simulink model "PosControl_HIL_advanced"  (R2023b)
settings: Solver=FixedStepDiscrete  StartTime=0.0  StopTime=10.0  FixedStep=0.001  RelTol=1e-3
InitFcn:
  | Init_control
values from neighbouring files (symbols this model uses):
  DEG2RAD = 0.0174533    [Init_control.m]
  MAX_CONTROL_ANGLE_RATE_PITCH = 220    [Init_control.m]
  MAX_CONTROL_ANGLE_RATE_ROLL = 220    [Init_control.m]
  MAX_CONTROL_VELOCITY_XY = 5    [Init_control.m]
  MAX_CONTROL_VELOCITY_Z = 3    [Init_control.m]
  Saturation_I_az = 5    [Init_control.m]
undefined symbols (not defined in the file or in its folder): DiscIntNeverNeededParam
libraries: simulink x7, pixhawk_slib_uORB_RW x5, pixhawk_slib_sensors_actuators x4
(part 1 of 2)
settings Model: Creator=wsh  LastModifiedBy=02
settings SolverCC: AlgebraicLoopSolver=TrustRegion
settings DataIOCC: ReturnWorkspaceOutputs=off
settings OptimizationCC: DefaultParameterBehavior=Inlined  MaxStackSize=64  EfficientTunableParamExpr=on
settings DebuggingCC: ParameterTunabilityLossMsg=error  UnconnectedInputMsg=warning  UnconnectedOutputMsg=warning  UnconnectedLineMsg=warning  ArithmeticOperatorsInVariantConditions=warning
settings HardwareCC: ProdBitPerPointer=32  ProdBitPerSizeT=32  ProdBitPerPtrDiffT=32  ProdLargestAtomicInteger=Long  ProdLargestAtomicFloat=Double  ProdWordSize=32  ProdHWDeviceType=ARM Compatible->ARM Cortex
settings ModelReferenceCC: EnableRefExpFcnMdlSchedulingChecks=on
settings SFSimCC: SimUseLocalCustomCode=off  MATLABDynamicMemAlloc=off  CustomCodeUndefinedFunction=UseInterfaceOnly
settings RTWCC: Description=Embedded Coder  SystemTargetFile=ert.tlc  HardwareBoard=Pixhawk PX4  TLCOptions="-aInlineSetEventsForThisBaseRateFcn=TLC_FALSE -aSuppressMultiTaskScheduler=TLC_FALSE  -aRateBasedStepFcn=0"  TemplateMakefile=ert_default_tmf  GenerateReport=on  RTWUseLocalCustomCode=off  Toolchain=Pixhawk Toolchain  IncludeHyperlinkInReport=on  LaunchReport=on  GenerateTraceInfo=on  GenerateTraceReport=on  GenerateTraceReportSl=on  GenerateTraceReportSf=on  GenerateTraceReportEml=on
settings CodeAppCC: ForceParamTrailComments=on  IgnoreCustomStorageClasses=off  OperatorAnnotations=on  SimulinkDataObjDesc=on  SFDataObjDesc=on  MATLABFcnDesc=on  InsertBlockDesc=on  StateflowObjectComments=on  MATLABSourceComments=on
settings ERTTargetCC: MultiwordLength=2048  ERTCustomFileTemplate=PX4_codertarget_file_process.tlc

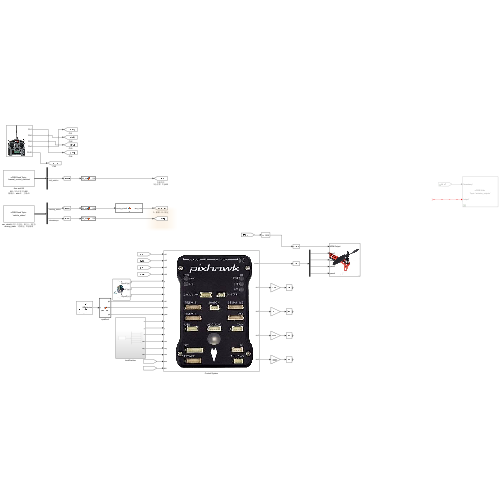
[thumbnail: Simulink's stored preview of the top-level diagram]
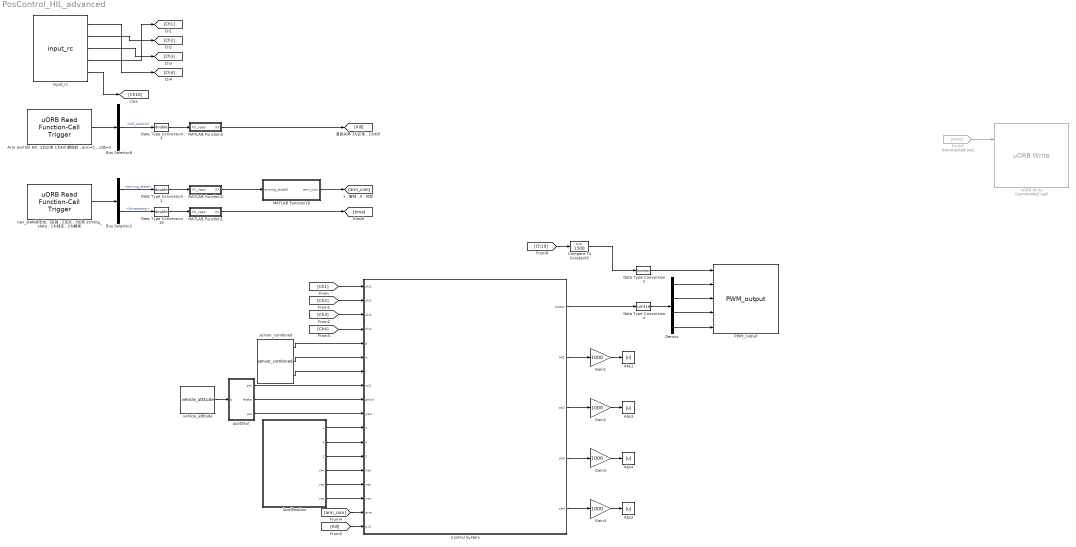
== system PosControl_HIL_advanced ==
  Abs{1..4} (4 alike) : Abs  SaturateOnIntegerOverflow=off
  Arm and Kill Kill：3为正常,1为Kill 解锁后，arm=1，上锁=3 : pixhawk_slib_uORB_RW/uORB Read Function-Call Trigger  uORB_Topic_str='manual_control_switches'  BusObjVar=Bus: manual_control_switches_SL  uORB_Interval=1  AsyncOutput=off  Fcn_call_select=Generate Function Call Signal  TaskName='Task1'  Poll_timeout=100  Ts=0.004
      settings: SourceProductName=Pixhawk Target Blocks
  Bus Selector2 : BusSelector  OutputSignals=arming_state,timestamp
  Bus Selector8 : BusSelector  OutputSignals=kill_switch
  Compare To Constant3 : simulink/Logic and Bit Operations/Compare To Constant  relop=>=  const=1500  OutDataTypeStr=boolean
  Control System : Subsystem
      mask Display: image('.\icon\pixhawk.png');
  Data Type Conversion1 : DataTypeConversion  OutDataTypeStr=double  SaturateOnIntegerOverflow=off  RndMeth=Floor
  Data Type Conversion19 : DataTypeConversion  OutDataTypeStr=double  SaturateOnIntegerOverflow=off  RndMeth=Floor
  Data Type Conversion2 : DataTypeConversion  OutDataTypeStr=boolean  SaturateOnIntegerOverflow=off  RndMeth=Floor
  Data Type Conversion3 : DataTypeConversion  OutDataTypeStr=double  SaturateOnIntegerOverflow=off  RndMeth=Floor
  Data Type Conversion4 : DataTypeConversion  OutDataTypeStr=uint16  SaturateOnIntegerOverflow=off  RndMeth=Floor
  Demux : Demux
  From6 : From  Commented=on  GotoTag=time
  Gain{1..4} (4 alike) : Gain  Gain=1000
  MATLAB Function1 : MATLAB Function  TreatAsAtomicUnit=on
  MATLAB Function18 : MATLAB Function  TreatAsAtomicUnit=on
  MATLAB Function2 : MATLAB Function  TreatAsAtomicUnit=on
  MATLAB Function3 : MATLAB Function  TreatAsAtomicUnit=on
  PWM_output : pixhawk_slib_sensors_actuators/PWM_output  Description=|  pub_outputs=on  pwm_rate=400Hz  show_pwm1=on  show_pwm5=off  show_pwm2=on  show_pwm6=off  show_pwm3=on  show_pwm7=off  show_pwm4=on  show_pwm8=off
      | This block allows the user to send the appropriate PWM signals out to the PX4 outputs.  
      | These are usually connected to the ESCs which control the motor speeds. 
      | In order for the flight control to arm (enable) the output from the software side, the ARM Output input must be held high (boolean TRUE).  
      | Only then will the PWM values be sent out the PX4 hardware ports.  
      | This is usually a function of the RC Tx in combination with other flight modes programmed in the Simulink model by the user.  
      | The block has 8 available ports (data type uint16) which can be selectively chosen.  
      | These correspond to the 8 PWM output ports on the px4fmu hardware.
      settings: SourceProductName=Pixhawk Target Blocks
  input_rc : pixhawk_slib_sensors_actuators/input_rc  Description=|  sampletime=0.004  channel1=on  channel2=on  channel3=on  channel4=on  channel5=off  channel6=off  channel7=off  channel8=off  channel9=off  channel10=on  channel11=off  channel12=off  channel13=off  channel14=off  channel15=off  channel16=off  channel17=off  channel18=off  ch_count=off  rssi=off  rc_failsafe=off  rc_lost=off  rc_inputsource=off
      | RC Input Block
      | 
      | This block provides user input control to the model.
      | It uses the input_rc uORB topic.
      | 
      | The user has the ability to choose which channels are available as outputs from this block and also some optional outputs. These include 
      | Channels 1 through 18
      | double data type indicating the PWM value from the controller 
      | measured pulse widths for each of the supported channels 
      | Channel Count 
      | uint32 data type of the number of channels which are detector by the PX4 
      | RC Failsafe 
      | boolean data types indicating that the RC Tx is sending the FailSafe signal (if equipped and properly setup) 
      | explicit failsafe flag: true on TX failure or TX out of range , false otherwise. 
      | Only the true state is reliable, as there are some (PPM) receivers on the market going into failsafe without telling us explicitly. 
      | RC Input Source 
      | Enumeration data type indicating which source the RC input is from. 
      | Valid values are found in the ENUM file: RC_INPUT_SOURCE_ENUM.m 
      |           Enumeration members for class 'RC_INPUT_SOURCE_ENUM':
      |           RCINPUT_SOURCE_UNKNOWN         (0)
      |           RCINPUT_SOURCE_PX4FMU_PPM      (1)
      |           RCINPUT_SOURCE_PX4IO_PPM       (2)
      |           RCINPUT_SOURCE_PX4IO_SPEKTRUM  (3)
      |           RCINPUT_SOURCE_PX4IO_SBUS      (4)
      |           RCINPUT_SOURCE_PX4IO_ST24      (5)
      |           RCINPUT_SOURCE_MAVLINK         (6)
      |           RCINPUT_SOURCE_QURT            (7)
      |           RCINPUT_SOURCE_PX4FMU_SPEKTRUM (8)
      |           RCINPUT_SOURCE_PX4FMU_SBUS     (9)
      |           RCINPUT_SOURCE_PX4FMU_ST24     (10)
      |           RCINPUT_SOURCE_PX4FMU_SUMD     (11)
      |           RCINPUT_SOURCE_PX4FMU_DSM      (12)
      |           RCINPUT_SOURCE_PX4IO_SUMD      (13)
      | 
      | RSSI - Receive signal strength index 
      | receive signal strength indicator (RSSI): < 0: Undefined, 0: no signal, 255: full reception 
      | RC Lost Connection 
      | boolean data type indicating RC receiver connection status 
      | True, if no frame has arrived in the expected time, false otherwise. 
      | True usally means that the receiver has been disconnected, but can also indicate a radio link loss on "stupid" systems. 
      | Will remain false, if a RX with failsafe option continues to transmit frames after a link loss. 
      |   
      | Sample Model: px4demo_input_rc.slx
      settings: SourceProductName=Pixhawk Target Blocks
  "localPosition " : Subsystem
  nav_state标志位: 1定高，2定点，3任务 arming_state：1为锁定，2为解锁 : pixhawk_slib_uORB_RW/uORB Read Function-Call Trigger  uORB_Topic_str='vehicle_status'  BusObjVar=Bus: vehicle_status_SL  uORB_Interval=1  AsyncOutput=off  Fcn_call_select=Generate Function Call Signal  TaskName='Task1'  Poll_timeout=100  Ts=0.004
      settings: SourceProductName=Pixhawk Target Blocks
  quat2eul : MATLAB Function  TreatAsAtomicUnit=on
  sensor_combined : pixhawk_slib_sensors_actuators/sensor_combined  Description=|  sampletime=0.001  show_mag=off  show_acc=off  show_gyro=on  show_baro=off  show_ts=off
      | Sensor Combined Block
      | 
      | This block enables access to the various sensors available on the px4fmu-v2 hardware.  
      | The user can use these signals in the Simulink control model.  
      | The sample time needs to be provided in the mask dialog.  
      | Optional output ports can also be selected.  
      | Refer to the sample model: px4demo_attitude_control.slx
      | 
      | Signal definitions: 
      | Magnetometer (x,y,z) - single values – Magnetic field in NED body frame, in Gauss 
      | Accelerometer (x,y,z) - single values – Acceleration in NED body frame, in m/s^2 
      | Gyroscope (p,q,r) - single values – Angular velocity in radians per second 
      | Barometer (Altitude) - single value – Barometric pressure, already temperature compensated (millibars) 
      | RunTime (timestamp) - double value – Timestamp in microseconds since boot, from gyro 
      |   
      | The sensor_combined block needs to have the px4io service running on the PX4 hardware in order to get valid signal values.
      settings: SourceProductName=Pixhawk Target Blocks
  uORB Write : pixhawk_slib_uORB_RW/uORB Write  Commented=on  uORB_Topic_str='actuator_outputs'  BlockOutputCount=2  OutputBoolean_1=on  uORB_Param_Name1='timestamp'  uORB_Param_Name_DT1=double  VectorScalar_1=1  OutputBoolean_2=on  uORB_Param_Name2='output'  uORB_Param_Name_DT2=double  VectorScalar_2=16  OutputBoolean_3=off  uORB_Param_Name3='timestamp_time'  uORB_Param_Name_DT3=double  VectorScalar_3=1  OutputBoolean_4=off  uORB_Param_Name4='gyro_temp'  uORB_Param_Name_DT4=single  VectorScalar_4=3  OutputBoolean_5=off  uORB_Param_Name5='vel_ned_valid'  uORB_Param_Name_DT5=boolean  VectorScalar_5=1  Ts=-1  MsgSizeOf=0
      settings: SourceProductName=Pixhawk Target Blocks
  vehicle_attitude : pixhawk_slib_sensors_actuators/vehicle_attitude  Description=|  sampletime=0.001  show_r=off  show_p=off  show_y=off  show_q=on  show_ts=off
      | This block gives access to the running service that calculates the vehicle’s attitude.  A uORB topic (vehicle_attitude (attitude measurements)) publisher MUST be running in order for this block to provide valid signal values.  The available ones as of v1.3 are: 
      | attitude_estimator_ekf – EKF-Extended Kalman Filter for attitude estimation 
      | attitude_estimator_so3 – SO(3)-attitude estimation by using accelerometer, gyroscopes and magnetometer 
      | One of these MUST be running on the px4fmu in order for this block to return valid values.  Refer to the sample model: px4demo_attitude_control.slx. Attitude in NED (North-East-Down) body frame in SI units. 
      | Signal definitions: 
      | Roll – single value, Roll angle (rad, Tait-Bryan, NED) 
      | Pitch – single value, Pitch angle (rad, Tait-Bryan, NED) 
      | Yaw – single value, Yaw angle (rad, Tait-Bryan, NED) 
      | Quaternion (NED) – single(4) values (optional based on the uORB publisher)
      settings: SourceProductName=Pixhawk Target Blocks
  wires:
  sensor_combined/1 -> Control System/5(p)
  sensor_combined/3 -> Control System/7(r)
  sensor_combined/2 -> Control System/6(q)
  "localPosition "/1(x) -> Control System/11(x)
  "localPosition "/3(z) -> Control System/13(z)
  "localPosition "/4(vex) -> Control System/14(vex)
  "localPosition "/5(vey) -> Control System/15(vey)
  "localPosition "/6(vez) -> Control System/16(vez)
  vehicle_attitude/1 -> quat2eul/1(q)
  quat2eul/1(phi) -> Control System/8(roll)
  quat2eul/3(psi) -> Control System/10(yaw)
  quat2eul/2(theta) -> Control System/9(pitch)
  Bus Selector2/1 -> Data Type Conversion1/1  "<arming_state>"
  MATLAB Function18/1(arm_com) -> [arm_com]
  Data Type Conversion1/1 -> MATLAB Function2/1(XX_read)
  nav_state标志位: 1定高，2定点，3任务 arming_state：1为锁定，2为解锁/1 -> Bus Selector2/1
  MATLAB Function2/1(XX) -> MATLAB Function18/1(arming_state0)
  Bus Selector8/1 -> Data Type Conversion3/1  "<kill_switch>"
  Data Type Conversion3/1 -> MATLAB Function3/1(XX_read)
  Arm and Kill Kill：3为正常,1为Kill 解锁后，arm=1，上锁=3/1 -> Bus Selector8/1
  MATLAB Function3/1(XX) -> [Kill]
  input_rc/2 -> [Ch2]
  input_rc/3 -> [Ch3]
  [Ch1] -> Control System/1(ch1)
  [Ch2] -> Control System/2(ch2)
  [Ch3] -> Control System/3(ch3)
  [Ch4] -> Control System/4(ch4)
  [arm_com] -> Control System/17(arm)
  [Kill] -> Control System/18(Kill)
  "localPosition "/2(y) -> Control System/12(y)
  MATLAB Function1/1(XX) -> [time]
  Bus Selector2/2 -> Data Type Conversion19/1  "<timestamp>"
  Data Type Conversion19/1 -> MATLAB Function1/1(XX_read)
  Control System/2(ob1) -> Gain1/1
  Gain1/1 -> Abs1/1
  Control System/3(ob2) -> Gain2/1
  Control System/5(ob4) -> Gain4/1
  Gain2/1 -> Abs3/1
  Control System/4(ob3) -> Gain3/1
  Gain3/1 -> Abs4/1
  Gain4/1 -> Abs2/1
  input_rc/1 -> [Ch4]
  input_rc/4 -> [Ch1]
  Demux/1 -> PWM_output/2
  Data Type Conversion4/1 -> Demux/1
  Demux/2 -> PWM_output/3
  Demux/3 -> PWM_output/4
  Demux/4 -> PWM_output/5
  From6/1 -> uORB Write/1
  ? -> uORB Write/2
  Compare To Constant3/1 -> Data Type Conversion2/1
  Control System/1(motor) -> Data Type Conversion4/1
  Data Type Conversion2/1 -> PWM_output/1
  [Ch10] -> Compare To Constant3/1
  input_rc/5 -> [Ch10]

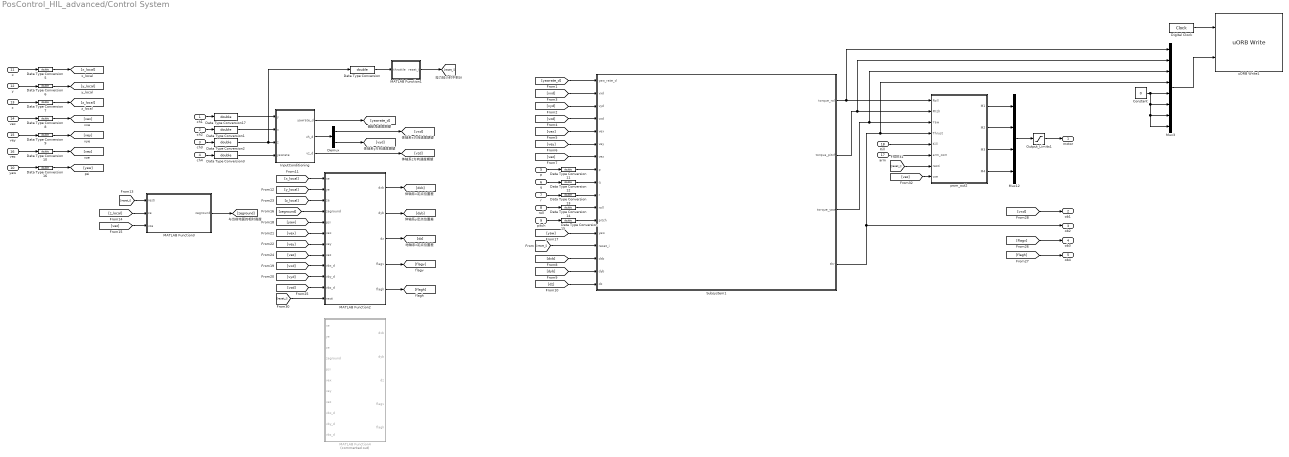
== system PosControl_HIL_advanced/Control System ==
  ch1 : Inport  OutDataTypeStr=uint16  PortDimensions=1
  ch2 : Inport  Port=2  OutDataTypeStr=uint16  PortDimensions=1
  ch3 : Inport  Port=3  OutDataTypeStr=uint16  PortDimensions=1
  ch4 : Inport  Port=4  OutDataTypeStr=uint16  PortDimensions=1
  p : Inport  Port=5  PortDimensions=1
  q : Inport  Port=6  PortDimensions=1
  r : Inport  Port=7  PortDimensions=1
  roll : Inport  Port=8  PortDimensions=1
  pitch : Inport  Port=9  PortDimensions=1
  yaw : Inport  Port=10  PortDimensions=1
  x : Inport  Port=11  PortDimensions=1
  y : Inport  Port=12  PortDimensions=1
  z : Inport  Port=13  PortDimensions=1
  vex : Inport  Port=14  PortDimensions=1
  vey : Inport  Port=15  PortDimensions=1
  vez : Inport  Port=16  PortDimensions=1
  arm : Inport  Port=17  PortDimensions=1
  Kill : Inport  Port=18  PortDimensions=1
  Constant : Constant  Value=0
  Data Type Conversion{,1..3,5..17} (17 alike) : DataTypeConversion  OutDataTypeStr=double  SaturateOnIntegerOverflow=off  RndMeth=Floor
  Demux : Demux  Outputs=2
  Digital Clock : DigitalClock  SampleTime=-1
  InputConditioning : Subsystem
  MATLAB Function1 : MATLAB Function  TreatAsAtomicUnit=on
  MATLAB Function2 : MATLAB Function  TreatAsAtomicUnit=on
  MATLAB Function3 : MATLAB Function  TreatAsAtomicUnit=on
  MATLAB Function4 : MATLAB Function  Commented=on  TreatAsAtomicUnit=on
  Mux12 : Mux
  Mux3 : Mux  Inputs=8
  Output_Limits1 : Saturate  UpperLimit=single(2000)  LowerLimit=single(1000)
  Subsystem1 : Subsystem
  pwm_out2 : MATLAB Function  SystemSampleTime=0.004
  uORB Write1 : pixhawk_slib_uORB_RW/uORB Write  uORB_Topic_str='rfly_px4'  BlockOutputCount=2  OutputBoolean_1=on  uORB_Param_Name1='timestamp'  uORB_Param_Name_DT1=double  VectorScalar_1=1  OutputBoolean_2=on  uORB_Param_Name2='control'  uORB_Param_Name_DT2=double  VectorScalar_2=8  OutputBoolean_3=off  uORB_Param_Name3='timestamp_time'  uORB_Param_Name_DT3=double  VectorScalar_3=1  OutputBoolean_4=off  uORB_Param_Name4='gyro_temp'  uORB_Param_Name_DT4=single  VectorScalar_4=3  OutputBoolean_5=off  uORB_Param_Name5='vel_ned_valid'  uORB_Param_Name_DT5=boolean  VectorScalar_5=1  Ts=-1  MsgSizeOf=0
      settings: SourceProductName=Pixhawk Target Blocks
  motor : Outport  VectorParamsAs1DForOutWhenUnconnected=off
  ob1 : Outport  Port=2  VectorParamsAs1DForOutWhenUnconnected=off
  ob2 : Outport  Port=3  VectorParamsAs1DForOutWhenUnconnected=off
  ob3 : Outport  Port=4  VectorParamsAs1DForOutWhenUnconnected=off
  ob4 : Outport  Port=5  VectorParamsAs1DForOutWhenUnconnected=off
  wires:
  roll/1 -> Data Type Conversion14/1
  pitch/1 -> Data Type Conversion15/1
  p/1 -> Data Type Conversion11/1
  q/1 -> Data Type Conversion12/1
  r/1 -> Data Type Conversion13/1
  MATLAB Function1/1(reset_i) -> [reset_i]
  yaw/1 -> Data Type Conversion16/1
  x/1 -> Data Type Conversion5/1
  z/1 -> Data Type Conversion7/1
  ch1/1 -> Data Type Conversion17/1
  InputConditioning/2(vh_d) -> Demux/1
  Data Type Conversion/1 -> MATLAB Function1/1(throttle)
  Data Type Conversion11/1 -> Subsystem1/8(p)
  Data Type Conversion12/1 -> Subsystem1/9(q)
  Data Type Conversion13/1 -> Subsystem1/10(r)
  Data Type Conversion14/1 -> Subsystem1/11(roll)
  Data Type Conversion15/1 -> Subsystem1/12(pitch)
  [reset_i] -> Subsystem1/14(reset_i)
  ch2/1 -> Data Type Conversion1/1
  ch4/1 -> Data Type Conversion3/1
  Data Type Conversion3/1 -> InputConditioning/4("yawrate ")
  ch3/1 -> Data Type Conversion2/1
  Data Type Conversion2/1 -> Data Type Conversion/1, InputConditioning/3(z)
  Data Type Conversion17/1 -> InputConditioning/1(y)
  Data Type Conversion1/1 -> InputConditioning/2(x)
  InputConditioning/1(yawrate_d) -> [yawrate_d]
  [yawrate_d] -> Subsystem1/1(yaw_rate_d)
  Demux/1 -> [vxd]
  Demux/2 -> [vyd]
  [vxd] -> Subsystem1/2(vxd)
  [vyd] -> Subsystem1/3(vyd)
  InputConditioning/3(vz_d) -> [vzd]
  [vzd] -> Subsystem1/4(vzd)
  Data Type Conversion5/1 -> [x_local]
  y/1 -> Data Type Conversion6/1
  Data Type Conversion6/1 -> [y_local]
  Data Type Conversion7/1 -> [z_local]
  pwm_out2/4(M4) -> Mux12/4
  pwm_out2/2(M2) -> Mux12/2
  Mux12/1 -> Output_Limits1/1
  Output_Limits1/1 -> motor/1
  pwm_out2/3(M3) -> Mux12/3
  pwm_out2/1(M1) -> Mux12/1
  arm/1 -> pwm_out2/6(arm_com)
  Kill/1 -> pwm_out2/5(Kill)
  [x_local] -> MATLAB Function2/1(xe)
  [y_local] -> MATLAB Function2/2(ye)
  [zeground] -> MATLAB Function2/4(zeground)
  MATLAB Function3/1(zeground) -> [zeground]
  [reset_i] -> MATLAB Function3/1(resti)
  [z_local] -> MATLAB Function3/2(ze)
  [vez] -> MATLAB Function3/3(vze)
  vex/1 -> Data Type Conversion8/1
  vey/1 -> Data Type Conversion9/1
  vez/1 -> Data Type Conversion10/1
  Data Type Conversion8/1 -> [vex]
  Data Type Conversion9/1 -> [vey]
  Data Type Conversion10/1 -> [vez]
  Data Type Conversion16/1 -> [yaw]
  [yaw] -> Subsystem1/13(yaw)
  [yaw] -> MATLAB Function2/5(psi)
  [vxd] -> MATLAB Function2/9(vbx_d)
  [vyd] -> MATLAB Function2/10(vby_d)
  [vex] -> MATLAB Function2/6(vex)
  [vey] -> MATLAB Function2/7(vey)
  [z_local] -> MATLAB Function2/3(ze)
  [vez] -> MATLAB Function2/8(vez)
  [vzd] -> MATLAB Function2/11(vbz_d)
  MATLAB Function2/1(dxb) -> [dxb]
  MATLAB Function2/2(dyb) -> [dyb]
  MATLAB Function2/3(dz) -> [dz]
  [vez] -> Subsystem1/7(vez)
  [vex] -> Subsystem1/5(vex)
  [vey] -> Subsystem1/6(vey)
  Subsystem1/1(torque_roll) -> Mux3/1, pwm_out2/1(Roll)
  Subsystem1/2(torque_pitch) -> Mux3/2, pwm_out2/2(Pitch)
  Subsystem1/3(torque_yaw) -> Mux3/3, pwm_out2/3(Yaw)
  [vxd] -> ob1/1
  Subsystem1/4(thr) -> Mux3/4, pwm_out2/4(Thrust), ob2/1
  [flagv] -> ob3/1
  [flagh] -> ob4/1
  [dxb] -> Subsystem1/15(dxb)
  [dyb] -> Subsystem1/16(dyb)
  [dz] -> Subsystem1/17(dz)
  MATLAB Function2/4(flagv) -> [flagv]
  MATLAB Function2/5(flagh) -> [flagh]
  [reset_i] -> MATLAB Function2/12(resti)
  [reset_i] -> pwm_out2/7(resti)
  [vez] -> pwm_out2/8(vze)
  Mux3/1 -> uORB Write1/2
  Digital Clock/1 -> uORB Write1/1
  Constant/1 -> Mux3/8, Mux3/7, Mux3/6, Mux3/5

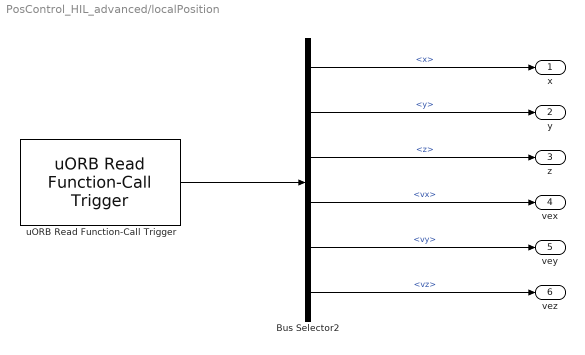
== system PosControl_HIL_advanced/localPosition  ==
  Bus Selector2 : BusSelector  OutputSignals=x,y,z,vx,vy,vz
  uORB Read Function-Call Trigger : pixhawk_slib_uORB_RW/uORB Read Function-Call Trigger  uORB_Topic_str='vehicle_local_position'  BusObjVar=Bus: vehicle_local_position_SL  uORB_Interval=1  AsyncOutput=off  Fcn_call_select=Generate Function Call Signal  TaskName='Task1'  Poll_timeout=100  Ts=0.004
      settings: SourceProductName=Pixhawk Target Blocks
  x : Outport  VectorParamsAs1DForOutWhenUnconnected=off
  y : Outport  Port=2  VectorParamsAs1DForOutWhenUnconnected=off
  z : Outport  Port=3  VectorParamsAs1DForOutWhenUnconnected=off
  vex : Outport  Port=4  VectorParamsAs1DForOutWhenUnconnected=off
  vey : Outport  Port=5  VectorParamsAs1DForOutWhenUnconnected=off
  vez : Outport  Port=6  VectorParamsAs1DForOutWhenUnconnected=off
  wires:
  uORB Read Function-Call Trigger/1 -> Bus Selector2/1
  Bus Selector2/6 -> vez/1  "<vz>"
  Bus Selector2/5 -> vey/1  "<vy>"
  Bus Selector2/4 -> vex/1  "<vx>"
  Bus Selector2/1 -> x/1  "<x>"
  Bus Selector2/2 -> y/1  "<y>"
  Bus Selector2/3 -> z/1  "<z>"

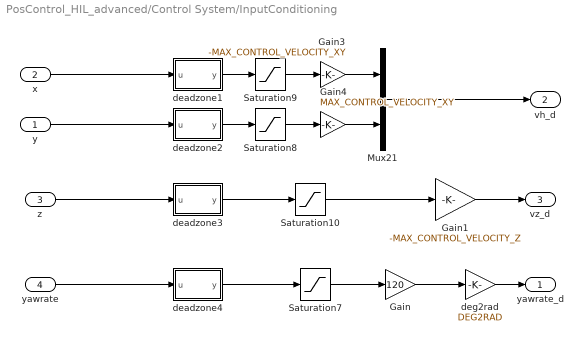
== system PosControl_HIL_advanced/Control System/InputConditioning ==
  y : Inport
  x : Inport  Port=2
  z : Inport  Port=3
  "yawrate " : Inport  Port=4
  Gain : Gain  Gain=120
  Gain1 : Gain  Gain=-MAX_CONTROL_VELOCITY_Z  OutDataTypeStr=Inherit: Inherit via back propagation
  Gain3 : Gain  Gain=-MAX_CONTROL_VELOCITY_XY  OutDataTypeStr=Inherit: Inherit via back propagation
  Gain4 : Gain  Gain=MAX_CONTROL_VELOCITY_XY  OutDataTypeStr=Inherit: Inherit via back propagation
  Mux21 : Mux  Inputs=2
  Saturation{7..10} (4 alike) : Saturate  UpperLimit=1  LowerLimit=-1
  deadzone1 : MATLAB Function  TreatAsAtomicUnit=on
  deadzone2 : MATLAB Function  TreatAsAtomicUnit=on
  deadzone3 : MATLAB Function  TreatAsAtomicUnit=on
  deadzone4 : MATLAB Function  TreatAsAtomicUnit=on
  deg2rad : Gain  Gain=DEG2RAD
  yawrate_d : Outport  VectorParamsAs1DForOutWhenUnconnected=off
  vh_d : Outport  Port=2  VectorParamsAs1DForOutWhenUnconnected=off
  vz_d : Outport  Port=3  VectorParamsAs1DForOutWhenUnconnected=off
  wires:
  Saturation10/1 -> Gain1/1
  Saturation7/1 -> Gain/1
  Mux21/1 -> vh_d/1
  deadzone3/1(y) -> Saturation10/1
  deadzone4/1(y) -> Saturation7/1
  Gain/1 -> deg2rad/1
  Gain1/1 -> vz_d/1
  z/1 -> deadzone3/1(u)
  "yawrate "/1 -> deadzone4/1(u)
  deadzone1/1(y) -> Saturation9/1
  Saturation9/1 -> Gain3/1
  x/1 -> deadzone1/1(u)
  Gain3/1 -> Mux21/1
  Saturation8/1 -> Gain4/1
  deadzone2/1(y) -> Saturation8/1
  y/1 -> deadzone2/1(u)
  Gain4/1 -> Mux21/2
  deg2rad/1 -> yawrate_d/1

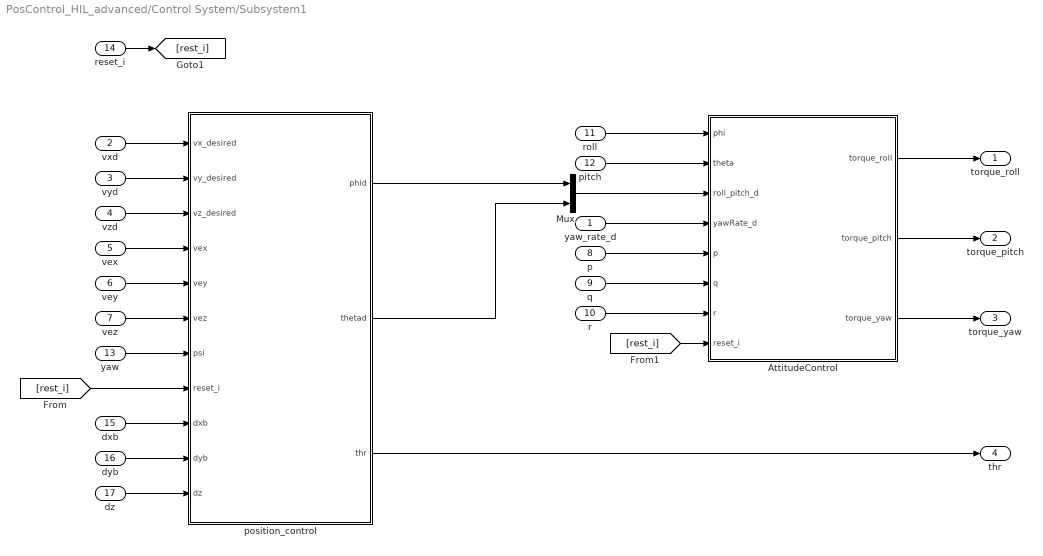
== system PosControl_HIL_advanced/Control System/Subsystem1 ==
  yaw_rate_d : Inport
  vxd : Inport  Port=2
  vyd : Inport  Port=3
  vzd : Inport  Port=4
  vex : Inport  Port=5
  vey : Inport  Port=6
  vez : Inport  Port=7
  p : Inport  Port=8  PortDimensions=1
  q : Inport  Port=9  PortDimensions=1
  r : Inport  Port=10  PortDimensions=1
  roll : Inport  Port=11  PortDimensions=1
  pitch : Inport  Port=12  PortDimensions=1
  yaw : Inport  Port=13
  reset_i : Inport  Port=14
  dxb : Inport  Port=15
  dyb : Inport  Port=16
  dz : Inport  Port=17
  AttitudeControl : Subsystem
  Mux : Mux  Inputs=2
  position_control : Subsystem
  torque_roll : Outport  VectorParamsAs1DForOutWhenUnconnected=off
  torque_pitch : Outport  Port=2  VectorParamsAs1DForOutWhenUnconnected=off
  torque_yaw : Outport  Port=3  VectorParamsAs1DForOutWhenUnconnected=off
  thr : Outport  Port=4  VectorParamsAs1DForOutWhenUnconnected=off
  wires:
  AttitudeControl/1(torque_roll) -> torque_roll/1
  pitch/1 -> AttitudeControl/2(theta)
  q/1 -> AttitudeControl/6(q)
  roll/1 -> AttitudeControl/1(phi)
  AttitudeControl/3(torque_yaw) -> torque_yaw/1
  r/1 -> AttitudeControl/7(r)
  AttitudeControl/2(torque_pitch) -> torque_pitch/1
  p/1 -> AttitudeControl/5(p)
  Mux/1 -> AttitudeControl/3(roll_pitch_d)
  position_control/1(phid) -> Mux/1
  yaw_rate_d/1 -> AttitudeControl/4(yawRate_d)
  position_control/2(thetad) -> Mux/2
  position_control/3(thr) -> thr/1
  vxd/1 -> position_control/1(vx_desired)
  vyd/1 -> position_control/2(vy_desired)
  vzd/1 -> position_control/3(vz_desired)
  vex/1 -> position_control/4(vex)
  vey/1 -> position_control/5(vey)
  vez/1 -> position_control/6(vez)
  yaw/1 -> position_control/7(psi)
  reset_i/1 -> [rest_i]
  [rest_i] -> position_control/8(reset_i)
  [rest_i] -> AttitudeControl/8(reset_i)
  dxb/1 -> position_control/9(dxb)
  dyb/1 -> position_control/10(dyb)
  dz/1 -> position_control/11(dz)

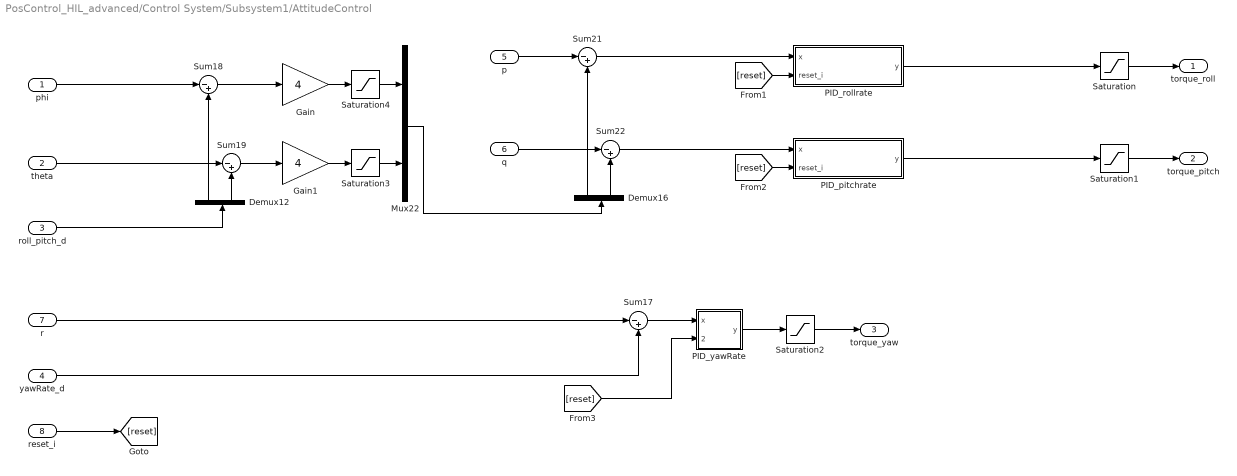
== system PosControl_HIL_advanced/Control System/Subsystem1/AttitudeControl ==
  phi : Inport
  theta : Inport  Port=2
  roll_pitch_d : Inport  Port=3
  yawRate_d : Inport  Port=4
  p : Inport  Port=5
  q : Inport  Port=6
  r : Inport  Port=7
  reset_i : Inport  Port=8
  Demux12 : Demux  Outputs=2
  Demux16 : Demux  Outputs=2
  Gain : Gain  Gain=4
  Gain1 : Gain  Gain=4
  Mux22 : Mux  Inputs=2
  PID_pitchrate : Subsystem
  PID_rollrate : Subsystem
  PID_yawRate : Subsystem
  Saturation : Saturate  UpperLimit=0.3  LowerLimit=-0.3
  Saturation1 : Saturate  UpperLimit=0.3  LowerLimit=-0.3
  Saturation2 : Saturate  UpperLimit=0.2  LowerLimit=-0.2
  Saturation3 : Saturate  UpperLimit=MAX_CONTROL_ANGLE_RATE_PITCH  LowerLimit=-MAX_CONTROL_ANGLE_RATE_PITCH
  Saturation4 : Saturate  UpperLimit=MAX_CONTROL_ANGLE_RATE_ROLL  LowerLimit=-MAX_CONTROL_ANGLE_RATE_ROLL
  Sum{17..19,21..22} (5 alike) : Sum  Inputs=|-+
  torque_roll : Outport  VectorParamsAs1DForOutWhenUnconnected=off
  torque_pitch : Outport  Port=2  VectorParamsAs1DForOutWhenUnconnected=off
  torque_yaw : Outport  Port=3  VectorParamsAs1DForOutWhenUnconnected=off
  wires:
  r/1 -> Sum17/1
  Sum19/1 -> Gain1/1
  Gain1/1 -> Saturation3/1
  Gain/1 -> Saturation4/1
  roll_pitch_d/1 -> Demux12/1
  Demux12/1 -> Sum18/2
  Demux12/2 -> Sum19/2
  phi/1 -> Sum18/1
  theta/1 -> Sum19/1
  Sum18/1 -> Gain/1
  Sum22/1 -> PID_pitchrate/1(x)
  Sum17/1 -> PID_yawRate/1(x)
  p/1 -> Sum21/1
  q/1 -> Sum22/1
  Sum21/1 -> PID_rollrate/1(x)
  Demux16/1 -> Sum21/2
  PID_pitchrate/1(y) -> Saturation1/1
  PID_rollrate/1(y) -> Saturation/1
  PID_yawRate/1(y) -> Saturation2/1
  yawRate_d/1 -> Sum17/2
  reset_i/1 -> [reset]
  [reset] -> PID_yawRate/2(reset_i)
  Saturation/1 -> torque_roll/1
  Saturation1/1 -> torque_pitch/1
  Saturation2/1 -> torque_yaw/1
  Mux22/1 -> Demux16/1
  Saturation4/1 -> Mux22/1
  Saturation3/1 -> Mux22/2
  Demux16/2 -> Sum22/2
  [reset] -> PID_rollrate/2(reset_i)
  [reset] -> PID_pitchrate/2(reset_i)

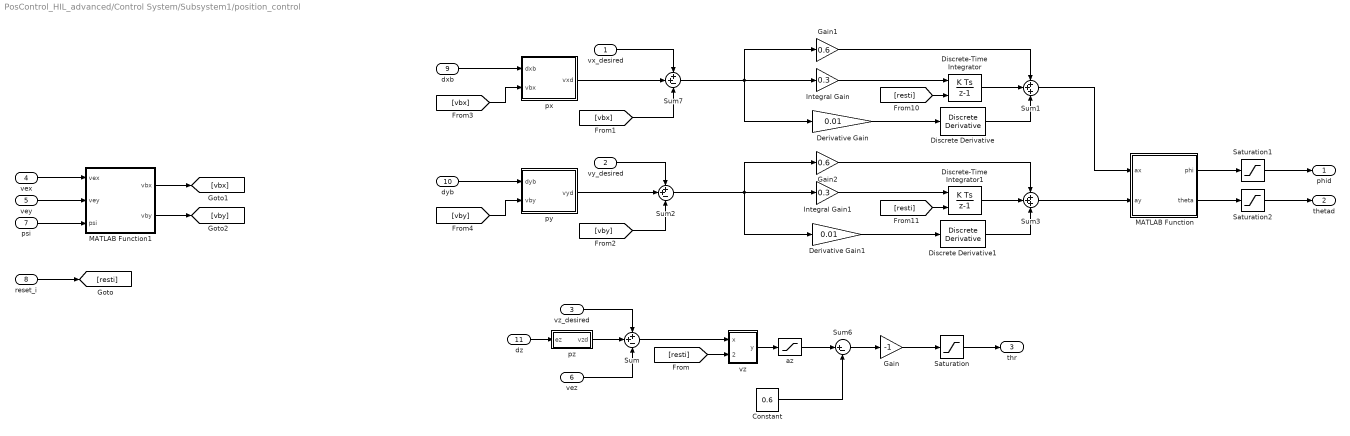
== system PosControl_HIL_advanced/Control System/Subsystem1/position_control ==
  vx_desired : Inport
  vy_desired : Inport  Port=2
  vz_desired : Inport  Port=3
  vex : Inport  Port=4
  vey : Inport  Port=5
  vez : Inport  Port=6
  psi : Inport  Port=7
  reset_i : Inport  Port=8
  dxb : Inport  Port=9
  dyb : Inport  Port=10
  dz : Inport  Port=11
  Constant : Constant  Value=0.6
  Derivative Gain : Gain  DisableCoverage=on  Gain=0.01
  Derivative Gain1 : Gain  DisableCoverage=on  Gain=0.01
  Discrete Derivative : simulink/Discrete/Discrete Derivative  gainval=1.0  ICPrevScaledInput=0.0  OutMin=[]  OutMax=[]  OutDataType=fixdt(1, 16)  OutScaling=2^-10  DoSatur=off
  Discrete Derivative1 : simulink/Discrete/Discrete Derivative  gainval=1.0  ICPrevScaledInput=0.0  OutMin=[]  OutMax=[]  OutDataType=fixdt(1, 16)  OutScaling=2^-10  DoSatur=off
  Discrete-Time Integrator : DiscreteIntegrator  ExternalReset=level  SampleTime=0.004  LimitOutput=on  UpperSaturationLimit=3.43  LowerSaturationLimit=-3.43  ICPrevOutput=DiscIntNeverNeededParam  ICPrevScaledInput=DiscIntNeverNeededParam
  Discrete-Time Integrator1 : DiscreteIntegrator  ExternalReset=level  SampleTime=0.004  LimitOutput=on  UpperSaturationLimit=3.43  LowerSaturationLimit=-3.43  ICPrevOutput=DiscIntNeverNeededParam  ICPrevScaledInput=DiscIntNeverNeededParam
  Gain : Gain  Gain=-1
  Gain1 : Gain  Gain=0.6
  Gain2 : Gain  Gain=0.6
  Integral Gain : Gain  DisableCoverage=on  Gain=0.3
  Integral Gain1 : Gain  DisableCoverage=on  Gain=0.3
  MATLAB Function : MATLAB Function  TreatAsAtomicUnit=on
  MATLAB Function1 : MATLAB Function  TreatAsAtomicUnit=on
  Saturation : Saturate  UpperLimit=0.85  LowerLimit=0
  Saturation1 : Saturate  UpperLimit=10/57.3  LowerLimit=-10/57.3
  Saturation2 : Saturate  UpperLimit=10/57.3  LowerLimit=-10/57.3
  Sum : Sum  Inputs=++-
  Sum1 : Sum  Inputs=+++
  Sum2 : Sum  Inputs=++-
  Sum3 : Sum  Inputs=+++
  Sum6 : Sum  Inputs=|+-
  Sum7 : Sum  Inputs=++-
  az : Saturate  UpperLimit=0.35  LowerLimit=-0.35
  px : Subsystem
  py : Subsystem
  pz : Subsystem
  "vz " : Subsystem
  phid : Outport  VectorParamsAs1DForOutWhenUnconnected=off
  thetad : Outport  Port=2  VectorParamsAs1DForOutWhenUnconnected=off
  thr : Outport  Port=3  VectorParamsAs1DForOutWhenUnconnected=off
  wires:
  Saturation/1 -> thr/1
  Gain/1 -> Saturation/1
  Sum6/1 -> Gain/1
  "vz "/1(y) -> az/1
  Constant/1 -> Sum6/2
  Sum/1 -> "vz "/1(x)
  vez/1 -> Sum/3
  vy_desired/1 -> Sum2/1
  pz/1(vzd) -> Sum/2
  vz_desired/1 -> Sum/1
  px/1(vxd) -> Sum7/2
  Saturation1/1 -> phid/1
  Saturation2/1 -> thetad/1
  vx_desired/1 -> Sum7/1
  py/1(vyd) -> Sum2/2
  MATLAB Function/1(phi) -> Saturation1/1
  MATLAB Function/2(theta) -> Saturation2/1
  az/1 -> Sum6/1
  MATLAB Function1/1(vbx) -> [vbx]
  MATLAB Function1/2(vby) -> [vby]
  vex/1 -> MATLAB Function1/1(vex)
  vey/1 -> MATLAB Function1/2(vey)
  [vbx] -> Sum7/3
  [vby] -> Sum2/3
  dyb/1 -> py/1(dyb)
  dz/1 -> pz/1(ez)
  psi/1 -> MATLAB Function1/3(psi)
  Sum7/1 -> Gain1/1, Integral Gain/1, Derivative Gain/1
  Integral Gain/1 -> Discrete-Time Integrator/1
  Discrete-Time Integrator/1 -> Sum1/2
  Derivative Gain/1 -> Discrete Derivative/1
  Gain1/1 -> Sum1/1
  Discrete Derivative/1 -> Sum1/3
  [resti] -> Discrete-Time Integrator/2
  reset_i/1 -> [resti]
  Sum1/1 -> MATLAB Function/1(ax)
  Sum3/1 -> MATLAB Function/2(ay)
  Gain2/1 -> Sum3/1
  Discrete-Time Integrator1/1 -> Sum3/2
  Integral Gain1/1 -> Discrete-Time Integrator1/1
  Derivative Gain1/1 -> Discrete Derivative1/1
  Discrete Derivative1/1 -> Sum3/3
  Sum2/1 -> Gain2/1, Integral Gain1/1, Derivative Gain1/1
  [resti] -> Discrete-Time Integrator1/2
  [resti] -> "vz "/2(reset_i)
  dxb/1 -> px/1(dxb)
  [vbx] -> px/2(vbx)
  [vby] -> py/2(vby)

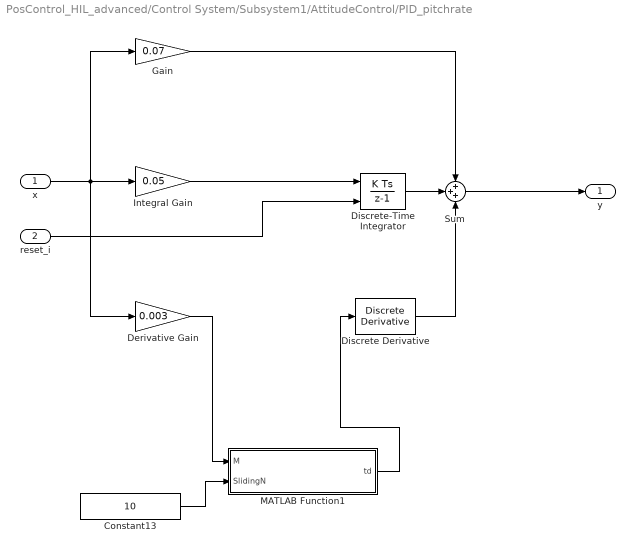
== system PosControl_HIL_advanced/Control System/Subsystem1/AttitudeControl/PID_pitchrate ==
  x : Inport
  reset_i : Inport  Port=2
  Constant13 : Constant  Value=10
  Derivative Gain : Gain  DisableCoverage=on  Gain=0.003  ParamMin=-100  ParamMax=100  OutMin=-100  OutMax=100
  Discrete Derivative : simulink/Discrete/Discrete Derivative  gainval=1.0  ICPrevScaledInput=0.0  OutMin=[]  OutMax=[]  OutDataType=fixdt(1, 16)  OutScaling=2^-10  DoSatur=off
  Discrete-Time Integrator : DiscreteIntegrator  ExternalReset=level  SampleTime=-1  LimitOutput=on  UpperSaturationLimit=0.1  LowerSaturationLimit=-0.1  ICPrevOutput=DiscIntNeverNeededParam  ICPrevScaledInput=DiscIntNeverNeededParam
  Gain : Gain  Gain=0.07
  Integral Gain : Gain  DisableCoverage=on  Gain=0.05
  MATLAB Function1 : MATLAB Function  TreatAsAtomicUnit=on
  Sum : Sum  Inputs=+++
  y : Outport  InitialOutput=0  VectorParamsAs1DForOutWhenUnconnected=off
  wires:
  x/1 -> Gain/1, Integral Gain/1, Derivative Gain/1
  Integral Gain/1 -> Discrete-Time Integrator/1
  Gain/1 -> Sum/1
  Sum/1 -> y/1
  Discrete Derivative/1 -> Sum/3
  Discrete-Time Integrator/1 -> Sum/2
  reset_i/1 -> Discrete-Time Integrator/2
  MATLAB Function1/1(td) -> Discrete Derivative/1
  Derivative Gain/1 -> MATLAB Function1/1(M)
  Constant13/1 -> MATLAB Function1/2(SlidingN)

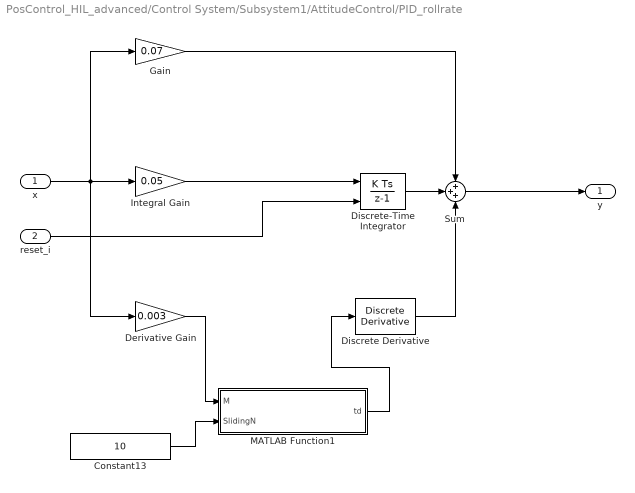
== system PosControl_HIL_advanced/Control System/Subsystem1/AttitudeControl/PID_rollrate ==
  x : Inport
  reset_i : Inport  Port=2
  Constant13 : Constant  Value=10
  Derivative Gain : Gain  DisableCoverage=on  Gain=0.003  ParamMin=-100  ParamMax=100  OutMin=-100  OutMax=100
  Discrete Derivative : simulink/Discrete/Discrete Derivative  gainval=1.0  ICPrevScaledInput=0.0  OutMin=[]  OutMax=[]  OutDataType=fixdt(1, 16)  OutScaling=2^-10  DoSatur=off
  Discrete-Time Integrator : DiscreteIntegrator  ExternalReset=level  SampleTime=-1  LimitOutput=on  UpperSaturationLimit=0.1  LowerSaturationLimit=-0.1  ICPrevOutput=DiscIntNeverNeededParam  ICPrevScaledInput=DiscIntNeverNeededParam
  Gain : Gain  Gain=0.07
  Integral Gain : Gain  DisableCoverage=on  Gain=0.05
  MATLAB Function1 : MATLAB Function  TreatAsAtomicUnit=on
  Sum : Sum  Inputs=+++
  y : Outport  InitialOutput=0  VectorParamsAs1DForOutWhenUnconnected=off
  wires:
  x/1 -> Gain/1, Integral Gain/1, Derivative Gain/1
  Integral Gain/1 -> Discrete-Time Integrator/1
  Gain/1 -> Sum/1
  Sum/1 -> y/1
  Discrete Derivative/1 -> Sum/3
  Discrete-Time Integrator/1 -> Sum/2
  reset_i/1 -> Discrete-Time Integrator/2
  Constant13/1 -> MATLAB Function1/2(SlidingN)
  Derivative Gain/1 -> MATLAB Function1/1(M)
  MATLAB Function1/1(td) -> Discrete Derivative/1

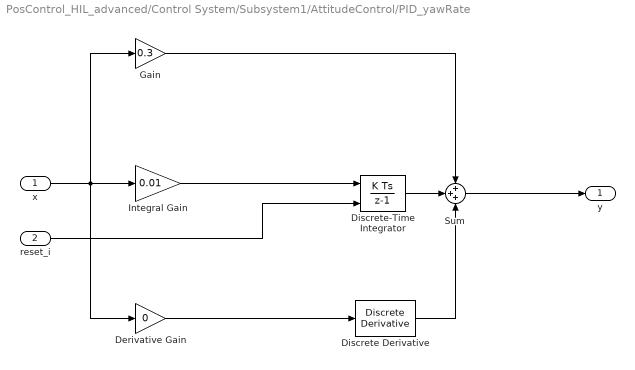
== system PosControl_HIL_advanced/Control System/Subsystem1/AttitudeControl/PID_yawRate ==
  x : Inport
  reset_i : Inport  Port=2
  Derivative Gain : Gain  DisableCoverage=on  Gain=0  ParamMin=-100  ParamMax=100  OutMin=-100  OutMax=100
  Discrete Derivative : simulink/Discrete/Discrete Derivative  gainval=1.0  ICPrevScaledInput=0.0  OutMin=[]  OutMax=[]  OutDataType=fixdt(1, 16)  OutScaling=2^-10  DoSatur=off
  Discrete-Time Integrator : DiscreteIntegrator  ExternalReset=level  SampleTime=-1  LimitOutput=on  UpperSaturationLimit=0.1  LowerSaturationLimit=-0.1  ICPrevOutput=DiscIntNeverNeededParam  ICPrevScaledInput=DiscIntNeverNeededParam
  Gain : Gain  Gain=0.3
  Integral Gain : Gain  DisableCoverage=on  Gain=0.01
  Sum : Sum  Inputs=+++
  y : Outport  InitialOutput=0  VectorParamsAs1DForOutWhenUnconnected=off
  wires:
  x/1 -> Derivative Gain/1, Integral Gain/1, Gain/1
  Integral Gain/1 -> Discrete-Time Integrator/1
  Derivative Gain/1 -> Discrete Derivative/1
  Gain/1 -> Sum/1
  Sum/1 -> y/1
  Discrete Derivative/1 -> Sum/3
  Discrete-Time Integrator/1 -> Sum/2
  reset_i/1 -> Discrete-Time Integrator/2

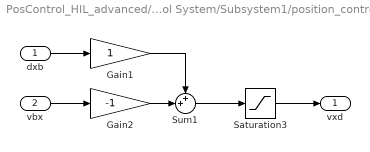
== system PosControl_HIL_advanced/Control System/Subsystem1/position_control/px ==
  dxb : Inport
  vbx : Inport  Port=2
  Gain1 : Gain
  Gain2 : Gain  Gain=-1
  Saturation3 : Saturate  UpperLimit=1  LowerLimit=-1
  Sum1 : Sum  Inputs=++|
  vxd : Outport  VectorParamsAs1DForOutWhenUnconnected=off
  wires:
  Sum1/1 -> Saturation3/1
  dxb/1 -> Gain1/1
  Saturation3/1 -> vxd/1
  vbx/1 -> Gain2/1
  Gain1/1 -> Sum1/1
  Gain2/1 -> Sum1/2

== system PosControl_HIL_advanced/Control System/Subsystem1/position_control/py ==
  dyb : Inport
  vby : Inport  Port=2
  Gain1 : Gain
  Gain2 : Gain  Gain=-1
  Saturation3 : Saturate  UpperLimit=1  LowerLimit=-1
  Sum1 : Sum  Inputs=++|
  vyd : Outport  VectorParamsAs1DForOutWhenUnconnected=off
  wires:
  Sum1/1 -> Saturation3/1
  dyb/1 -> Gain1/1
  Saturation3/1 -> vyd/1
  vby/1 -> Gain2/1
  Gain1/1 -> Sum1/1
  Gain2/1 -> Sum1/2

== system PosControl_HIL_advanced/Control System/Subsystem1/position_control/pz ==
  ez : Inport
  Gain1 : Gain
  Saturation3 : Saturate  UpperLimit=MAX_CONTROL_VELOCITY_Z  LowerLimit=-MAX_CONTROL_VELOCITY_Z
  vzd : Outport  VectorParamsAs1DForOutWhenUnconnected=off
  wires:
  ez/1 -> Gain1/1
  Saturation3/1 -> vzd/1
  Gain1/1 -> Saturation3/1

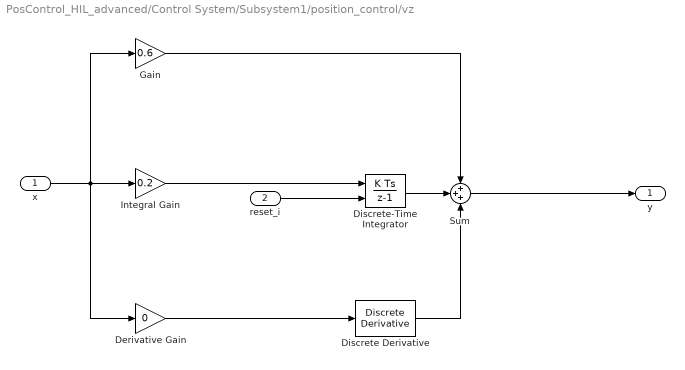
== system PosControl_HIL_advanced/Control System/Subsystem1/position_control/vz  ==
  x : Inport
  reset_i : Inport  Port=2
  Derivative Gain : Gain  DisableCoverage=on  Gain=0
  Discrete Derivative : simulink/Discrete/Discrete Derivative  gainval=1.0  ICPrevScaledInput=0.0  OutMin=[]  OutMax=[]  OutDataType=fixdt(1, 16)  OutScaling=2^-10  DoSatur=off
  Discrete-Time Integrator : DiscreteIntegrator  ExternalReset=level  SampleTime=0.004  LimitOutput=on  UpperSaturationLimit=Saturation_I_az  LowerSaturationLimit=-Saturation_I_az  ICPrevOutput=DiscIntNeverNeededParam  ICPrevScaledInput=DiscIntNeverNeededParam
  Gain : Gain  Gain=0.6
  Integral Gain : Gain  DisableCoverage=on  Gain=0.2
  Sum : Sum  Inputs=+++
  y : Outport  InitialOutput=0  VectorParamsAs1DForOutWhenUnconnected=off
  wires:
  Discrete-Time Integrator/1 -> Sum/2
  Discrete Derivative/1 -> Sum/3
  Sum/1 -> y/1
  Gain/1 -> Sum/1
  Derivative Gain/1 -> Discrete Derivative/1
  Integral Gain/1 -> Discrete-Time Integrator/1
  x/1 -> Derivative Gain/1, Integral Gain/1, Gain/1
  reset_i/1 -> Discrete-Time Integrator/2

== matlab function PosControl_HIL_advanced/Control System/Subsystem1/AttitudeControl/PID_rollrate/MATLAB Function1 ==
  settings: updateMethod=DISCRETE
  data: M input; SlidingN input; td output
function td = tdfilter(M, SlidingN)

persistent i array

if isempty(i)
    i=1;
end

if isempty(array)
    array = zeros(1,50);
end

array(i) = M;
i = i+1;

if i > SlidingN
    i = 1;
end

td = sum(array) / SlidingN;

== matlab function PosControl_HIL_advanced/quat2eul ==
  data: q input; phi output; theta output; psi output
function [phi,theta,psi] = quat2eul(q)
% Conversion from Quaternion to Euler angles based on the PX4 Firmware
% v1.6.5 release.
% 
% Quaternion -> DCM -> Euler Angles
% INPUT:
%   q: Quaternion vector of the format: (a + bi + cj + dk)
% OUTPUT:
%   [phi,theta,psi]: Euler angles in radians.
% 
 
    a = q(1);
    b = q(2);
    c = q(3);
    d = q(4);

    aSq = a*a;
    bSq = b*b;
    cSq = c*c;
    dSq = d*d;

    d_pi2 = pi/2;

    % quaternion_to_dcm
    dcm00 = aSq + bSq - cSq - dSq;
    % dcm01 = 2*(b*c - a*d);
    dcm02 = 2*(a*c + b*d);
    dcm10 = 2*(b*c + a*d);
    % dcm11 = aSq - bSq + cSq - dSq;
    dcm12 = 2*(c*d - a*b);
    dcm20 = 2*(b*d - a*c);
    dcm21 = 2*(a*b + c*d);
    dcm22 = aSq - bSq - cSq + dSq;

    % dcm_to_euler
    theta = asin(-dcm20);
    if abs(theta - d_pi2) < 1.0e-3
        phi = single(0.0);
        psi = atan2(dcm12, dcm02);
    elseif abs(theta + d_pi2) < 1.0e-3
        phi = single(0.0);
        psi = atan2(-dcm12, -dcm02);
    else
        phi = atan2(dcm21, dcm22);
        psi = atan2(dcm10, dcm00);
    end

end

== matlab function PosControl_HIL_advanced/Control System/Subsystem1/AttitudeControl/PID_pitchrate/MATLAB Function1 ==
  settings: updateMethod=DISCRETE
  data: M input; SlidingN input; td output
function td = tdfilter(M, SlidingN)

persistent i array

if isempty(i)
    i=1;
end

if isempty(array)
    array = zeros(1,50);
end

array(i) = M;
i = i+1;

if i > SlidingN
    i = 1;
end

td = sum(array) / SlidingN;

== matlab function PosControl_HIL_advanced/MATLAB Function2 ==
  data: XX_read input; XX output
function XX = fcn(XX_read)
if isnan(XX_read) 
    XX = 0;
else
    XX = XX_read;
end

== matlab function PosControl_HIL_advanced/MATLAB Function18 ==
  data: arming_state0 input; arm_com output
function arm_com = fcn(arming_state0) % 1为锁定，2为解锁
if arming_state0 > 1.5
    arm_com = 1;
else
    arm_com = 0;
end

== matlab function PosControl_HIL_advanced/MATLAB Function3 ==
  data: XX_read input; XX output
function XX = fcn(XX_read)
if isnan(XX_read) 
    XX = 0;
else
    XX = XX_read;
end

== matlab function PosControl_HIL_advanced/Control System/Subsystem1/position_control/MATLAB Function ==
  data: ax input; ay input; phi output; theta output
function [phi, theta] = fcn(ax, ay)
%Function description:
%  Convert the desired horizontal acceleration to the desired attitude angle
%Input:
%  eax, eaxy: desired horizontal acceleration
%  psi: yaw
%Output:
%  phi, theta: desired roll angle and desired pitch angle
g = 9.8;
phi = ay/g;
theta = -ax/g;

== matlab function PosControl_HIL_advanced/Control System/Subsystem1/position_control/MATLAB Function1 ==
  data: vex input; vey input; psi input; vbx output; vby output
function [vbx, vby] = fcn(vex, vey, psi)
%转为体轴系
vbx = sin(psi)*vey + cos(psi)*vex;
vby = cos(psi)*vey - sin(psi)*vex;

== matlab function PosControl_HIL_advanced/Control System/MATLAB Function2 ==
  data: xe input; ye input; ze input; zeground input; psi input; dxb output; dyb output; vex input; vey input; vez input; vbx_d input; vby_d input; vbz_d input; dz output; flagv output; flagh output; resti input
function [dxb, dyb, dz, flagv, flagh] = fcn(xe, ye, ze, zeground, psi, vex, vey, vez, vbx_d, vby_d, vbz_d, resti)
%转为体轴系
persistent xepos yepos zepos posflag_h posflag_v FFH FFV
if isempty(xepos)
    xepos = 0;
end
if isempty(yepos)
    yepos = 0;
end
if isempty(zepos)
    zepos = 0;
end
if isempty(posflag_h)
    posflag_h = 0;
end
if isempty(posflag_v)
    posflag_v = 0;
end
if isempty(FFH)
    FFH = 0;
end
if isempty(FFV)
    FFV = 0;
end

%% 水平方向定点处理
vtemp_h  = abs(vex)+abs(vey);          % 实时记录当前水平速度
vtempd_h = abs(vbx_d)+abs(vby_d);      % 实时记录当前期望的水平速度（遥控给的）
dxb=0;
dyb=0;

if vtempd_h >= 0.3
    dxb=0;
    dyb=0;                                                % 如果当前期望的水平速度大于0.1m/s（遥控给的），那就不做定点控制，posflag_h = 0
    posflag_h = 0;
    FFH = 0;                                              % 不做记录
end 

if vtemp_h < 0.3 && vtempd_h < 0.5 && FFH < 0.5           % 空中定点记录  
    xepos = xe;                                           % 则记录当前水平点
    yepos = ye;                                           
    posflag_h = 1;
    FFH = 1;                                              % 只记录一次
end  

if resti > 0.5 && abs(vez) < 0.1 % 在地面定点记录，这里不考虑FFH，如果只记录一次，万一有人把无人机位置移动了，那起飞就摔了
    xepos = xe;                                          
    yepos = ye;                                           
    posflag_h = 1;
end  

if posflag_h > 0.5 && FFH > 0.5
    dxb = sin(psi)*(yepos-ye) + cos(psi)*(xepos-xe);      % 输出dxb，dyb做定点控制
    dyb = cos(psi)*(yepos-ye) - sin(psi)*(xepos-xe);
end

flagh = posflag_h;

%% 垂直方向定点处理
vtemp_v = abs(vez);
vtempd_v = abs(vbz_d);
dz=0;

if vtempd_v >= 0.3
    dz=0;                                                % 如果当前期望的垂向速度大于0.1m/s，那就不做定点控制，posflag_h = 0
    posflag_v = 0;
    FFV = 0;
end 

if vtemp_v < 0.2 && vtempd_v < 0.3 && FFV < 0.5     % 空中定点记录  
    zepos = ze;                                           
    posflag_v = 1;
    FFV = 1;
end  

%if resti > 0.5 && abs(vez) < 0.1 % 在地面定点记录
%    zepos = ze;                                           
%    posflag_v = 1;
%end  
               
if posflag_v > 0.5 && FFV > 0.5                          % 如果posflag_v，说明记录了定点位置，则固定在位置点zepos
   dz = zepos-ze;                                        % 输出dz做定点控制
end

flagv = posflag_v;

end

% %% 如果离地高度小于0.8m，则不做定点处理
% if abs(zeground) < 0.8
%    dxb = 0;
%    dyb = 0;
%    dz = 0;
%    posflag_h = 0;
%    posflag_v = 0;
% end

== matlab function PosControl_HIL_advanced/Control System/MATLAB Function3 ==
  data: resti input; zeground output; ze input; vze input
function zeground = motorarm(resti, ze, vze)
persistent ze0
if isempty(ze0)
    ze0 = 0;
end

if resti > 0.5 && abs(vze) < 0.5 % 在地面
    ze0 = ze;
end

zeground = ze - ze0;

== matlab function PosControl_HIL_advanced/Control System/InputConditioning/deadzone1 ==
  data: u input; y output
function y = fcn(u)
%Function description:
%  Control the range of the remote control input from RCMin to RCMax, and
%  set a dead zone with a dead zone size of ±deadZone. The output y is
%  normalized to 0~1.You can get the RC calibration parameters in QGC.
RCMin = 1100;
RCMax = 1900;
RCMid = (RCMin + RCMax)/2;
deadZoneRate = 0.05;
deadZone = deadZoneRate*(RCMax - RCMin);
k = 1/(RCMax - RCMid - deadZone);
% saturation
if(u < RCMin)
    u = RCMin;
elseif(u > RCMax)
    u = RCMax;
end
% dead zone and normalize
 if(u > RCMid + deadZone)
    y = (u-RCMid - deadZone)*k;
 elseif(u < RCMid - deadZone)
     y = (u - RCMid + deadZone)*k;
 else
     y = 0;
 end

 end

== matlab function PosControl_HIL_advanced/Control System/InputConditioning/deadzone2 ==
  data: u input; y output
function y = fcn(u)
%Function description:
%  Control the range of the remote control input from RCMin to RCMax, and
%  set a dead zone with a dead zone size of ±deadZone. The output y is
%  normalized to 0~1.You can get the RC calibration parameters in QGC.
RCMin = 1100;
RCMax = 1900;
RCMid = (RCMin + RCMax)/2;
deadZoneRate = 0.05;
deadZone = deadZoneRate*(RCMax - RCMin);
k = 1/(RCMax - RCMid - deadZone);
% saturation
if(u < RCMin)
    u = RCMin;
elseif(u > RCMax)
    u = RCMax;
end
% dead zone and normalize
 if(u > RCMid + deadZone)
    y = (u-RCMid - deadZone)*k;
 elseif(u < RCMid - deadZone)
     y = (u - RCMid + deadZone)*k;
 else
     y = 0;
 end

 end

== matlab function PosControl_HIL_advanced/Control System/InputConditioning/deadzone3 ==
  data: u input; y output
function y = fcn(u)
%Function description:
%  Control the range of the remote control input from RCMin to RCMax, and
%  set a dead zone with a dead zone size of ±deadZone. The output y is
%  normalized to 0~1.You can get the RC calibration parameters in QGC.
RCMin = 1100;
RCMax = 1900;
RCMid = (RCMin + RCMax)/2;
deadZoneRate = 0.05;
deadZone = deadZoneRate*(RCMax - RCMin);
k = 1/(RCMax - RCMid - deadZone);
% saturation
if(u < RCMin)
    u = RCMin;
elseif(u > RCMax)
    u = RCMax;
end
% dead zone and normalize
 if(u > RCMid + deadZone)
    y = (u-RCMid - deadZone)*k;
 elseif(u < RCMid - deadZone)
     y = (u - RCMid + deadZone)*k;
 else
     y = 0;
 end

 end

== matlab function PosControl_HIL_advanced/Control System/MATLAB Function1 ==
  data: throttle input; reset_i output
function reset_i = fcn(throttle)
%Function description:
%  Reset Integral when throttle < 1250
if throttle < 1250
    reset_i = 1;
else
    reset_i = 0;
end

== matlab function PosControl_HIL_advanced/Control System/InputConditioning/deadzone4 ==
  data: u input; y output
function y = fcn(u)
%Function description:
%  Control the range of the remote control input from RCMin to RCMax, and
%  set a dead zone with a dead zone size of ±deadZone. The output y is
%  normalized to 0~1.You can get the RC calibration parameters in QGC.
RCMin = 1100;
RCMax = 1900;
RCMid = (RCMin + RCMax)/2;
deadZoneRate = 0.15;
deadZone = deadZoneRate*(RCMax - RCMin);
k = 1/(RCMax - RCMid - deadZone);
% saturation
if(u < RCMin)
    u = RCMin;
elseif(u > RCMax)
    u = RCMax;
end
% dead zone and normalize
 if(u > RCMid + deadZone)
    y = (u-RCMid - deadZone)*k;
 elseif(u < RCMid - deadZone)
     y = (u - RCMid + deadZone)*k;
 else
     y = 0;
 end

 end

== matlab function PosControl_HIL_advanced/Control System/MATLAB Function4 ==
  data: xe input; ye input; ze input; zeground input; psi input; dxb output; dyb output; vex input; vey input; vez input; vbx_d input; vby_d input; vbz_d input; dz output; flagv output; flagh output
function [dxb, dyb, dz, flagv, flagh] = fcn(xe, ye, ze, zeground, psi, vex, vey, vez, vbx_d, vby_d, vbz_d)
%转为体轴系
persistent xepos yepos zepos posflag_h posflag_v
if isempty(xepos)
    xepos = 0;
end
if isempty(yepos)
    yepos = 0;
end
if isempty(zepos)
    zepos = 0;
end
if isempty(posflag_h)
    posflag_h = 0;
end
if isempty(posflag_v)
    posflag_v = 0;
end

%% 水平方向定点处理
vtemp_h  = abs(vex)+abs(vey);          % 实时记录当前水平速度
vtempd_h = abs(vbx_d)+abs(vby_d);      % 实时记录当前期望的水平速度
dxb=0;
dyb=0;

if vtempd_h >= 0.1
    dxb=0;
    dyb=0;                                                % 如果当前期望的水平速度大于0.1m/s，那就不做定点控制，posflag_h = 0
    posflag_h = 0;                                         
end 

% if vtemp_h >= 0.2
%     dxb=0;
%     dyb=0;                                                
%     posflag_h = 0;                                      % 如果当前水平速度大于>0.2m/s，那也不做定点控制，posflag_h = 0
% end 

if vtemp_h < 0.2 && vtempd_h < 0.1 && posflag_h < 0.5     % 如果水平速度小于0.2m/s，且当前期望的水平速度小于0.1m/s，且还没有记录水平位置点
    xepos = xe;                                           % 则记录当前水平点
    yepos = ye;                                           % 并把posflag_h至1
    posflag_h = 1;                    
end                                                       % 情况1：vtemp_h继续减小，但由于posflag_h = 1，故xepos和yepos不做处理，因此xepos和yepos记录的是小于0.2m/s，但是最接近0.2m/s的位置点
                                                          % 情况2：vtemp_h大于0.2m/s，但vtempd_h < 0.1m/s，相当于有一个外部干扰，则xepos和yepos也不做处理，posflag_h = 1，即继续定位在干扰前的点
                      
if  posflag_h > 0.5                                       % 如果posflag_h = 1，说明记录了定点位置，则固定在位置点xepos与yepos
   % dxb = sin(psi)*(yepos-ye) + cos(psi)*(xepos-xe);      % 输出dxb，dyb做定点控制
   % dyb = cos(psi)*(yepos-ye) - sin(psi)*(xepos-xe); 
end

flagh = posflag_h;

%% 垂直方向定点处理
vtemp_v = abs(vez);
vtempd_v = abs(vbz_d);
dz=0;

if vtempd_v >= 0.1
    dz=0;                                                % 如果当前期望的垂向速度大于0.1m/s，那就不做定点控制，posflag_h = 0
    posflag_h = 0;                                         
end 

if vtemp_v < 0.2 && vtempd_v < 0.1 && posflag_v < 0.5    % 只要垂向速度小于0.2m/s，垂向杆不动，且还没有记录垂向位置点
    zepos = ze;                                          % 则记录当前垂向点
    posflag_v = 1;                                       % 并把posflag_v至1
end                                                      % 情况1：vtemp_v继续减小，但由于posflag_v = 1，故zepos不做处理，因此zepos记录的是小于0.2m/s，但是最接近0.2m/s的位置点
                                                         % 情况2：vtemp_v大于0.2m/s，但垂向杆不动，相当于有一个外部干扰，zepos不做处理
               
if posflag_v > 0.5                                       % 如果posflag_v，说明记录了定点位置，则固定在位置点zepos
   % dz = zepos-ze;                                       % 输出dz做定点控制
end

flagv = posflag_v;

end

% %% 如果离地高度小于0.8m，则不做定点处理
% if abs(zeground) < 0.8
%    dxb = 0;
%    dyb = 0;
%    dz = 0;
%    posflag_h = 0;
%    posflag_v = 0;
% end
